simulink model "disturbance_visualization"  (R2016b)
settings: Solver=VariableStepAuto  StartTime=0.0  StopTime=1  RelTol=1e-3
libraries: dspxfrm3 x1
settings Model: Creator=Jared  LastModifiedBy=Jared

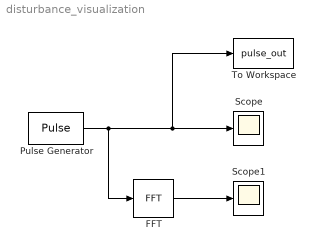
== system disturbance_visualization ==
  FFT : dspxfrm3/FFT  FFTImplementation=Auto  CompMethod=Table lookup  TableOpt=NEW  TableOptActive=Speed  BitRevOrder=off  Normalize=off  InheritFFTLength=on  FFTLength=64  WrapInput=on  roundingMode=Floor  overflowMode=off  firstCoeffDataTypeStr=Inherit: Same word length as input  firstCoeffLastDataTypeStr=Inherit: Same word length as input  outputMin=[]  outputMax=[]
  Pulse Generator : DiscretePulseGenerator  PulseType=Time based  Amplitude=-0.01  Period=1/44  PulseWidth=5
  Scope : Scope
  Scope1 : Scope
  To Workspace : ToWorkspace  VariableName=pulse_out  SaveFormat=Timeseries  SampleTime=-1
  wires:
  Pulse Generator/1 -> FFT/1, To Workspace/1, Scope/1
  FFT/1 -> Scope1/1
